simulink library "FAM_lab_scale_v3"  (R2024a)
settings: Solver=VariableStepAuto  StartTime=0.0  StopTime=10.0  RelTol=1e-3
undefined symbols (not defined in the file): FAM_elasticity, FAM_stretched_radius, FAM_unstretched_length, FAM_wall_thickness, fiber_angle_alpha, fiber_angle_alpha_unstr, hose_pump_force_enabled, hose_pump_max_stretch, hose_pump_throughFlow_adjust
settings Model: Creator=cmmcguir  LastModifiedBy=cmmcguir
settings RTWCC: GPUComputeCapability=3.5

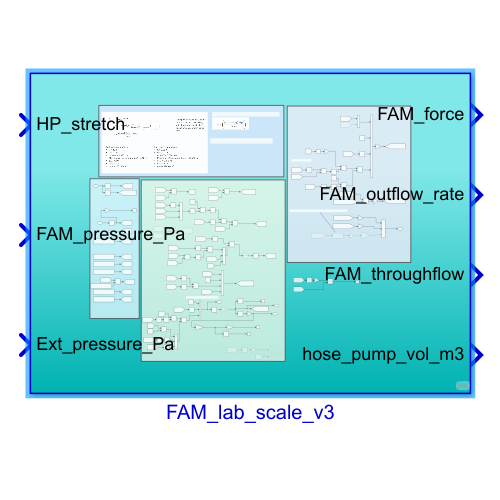
[thumbnail: Simulink's stored preview of the top-level diagram]
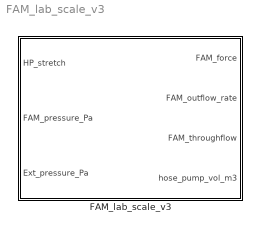
== system FAM_lab_scale_v3 ==
  FAM_lab_scale_v3 : Subsystem

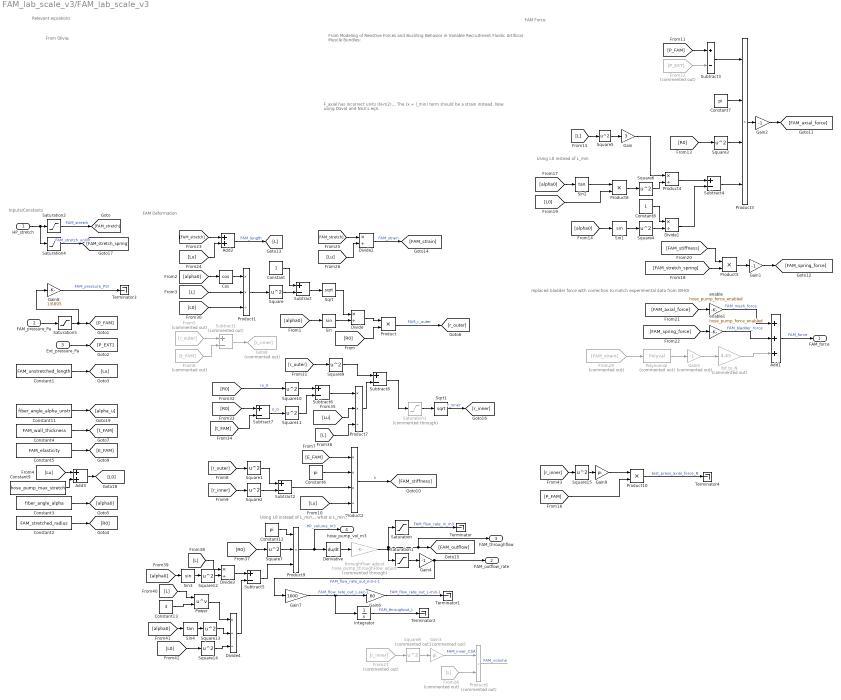
== system FAM_lab_scale_v3/FAM_lab_scale_v3 ==
  note: replaced bladder force with correction to match experimental data from WHOI
  note: F_axial has incorrect units (N-m2)... The (x + l_min) term should be a strain instead. Now using David and Nick's eqn.
  note: FAM Force
  note: Using L0 instead of L_min
  note: FAM Deformation
  note: Inputs/Constants
  note: Relevant equations
  note: From Modeling of Resistive Forces and Buckling Behavior in Variable Recruitment Fluidic Artificial Muscle Bundles:
  note: From Olivia:
  note: Using L0 instead of L_min... what is L_min?
  HP_stretch : Inport  Unit=m
  FAM_pressure_Pa : Inport  Port=2  Unit=Pa
  Ext_pressure_Pa : Inport  Port=3  Unit=Pa
  Add1 : Sum  Inputs=+++
  Add2 : Sum
  Add3 : Sum
  Constant : Constant
  Constant1 : Constant  Value=FAM_unstretched_length
  Constant11 : Constant  Value=fiber_angle_alpha_unstr
  Constant12 : Constant  Value=pi
  Constant13 : Constant  Value=3
  Constant2 : Constant  Value=FAM_stretched_radius
  Constant3 : Constant  Value=fiber_angle_alpha
  Constant4 : Constant  Value=FAM_wall_thickness
  Constant5 : Constant  Value=FAM_elasticity
  Constant6 : Constant  Value=pi
  Constant7 : Constant  Value=pi
  Constant8 : Constant
  Constant9 : Constant  Value=hose_pump_max_stretch
  Cos : Trigonometry  Operator=cos
  Derivative : Derivative
  Divide{,1..3} (4 alike) : Product  Inputs=*/
  Divide4 : Product  Inputs=*//
  From12 : From  Commented=on  GotoTag=P_EXT
  From27 : From  Commented=on  GotoTag=r_inner
  From28 : From  Commented=on  GotoTag=L
  From29 : From  Commented=on  GotoTag=FAM_strain
  From5 : From  Commented=on  GotoTag=r_outer
  From6 : From  Commented=on  GotoTag=t_FAM
  Gain : Gain  Gain=3
  Gain1 : Gain  Gain=-1
  Gain2 : Gain  Gain=-1
  Gain3 : Gain  Commented=on  Gain=pi
  Gain4 : Gain  Gain=-1
  Gain5 : Gain  Commented=on  Gain=-1
  Gain6 : Gain  Gain=60
  Gain7 : Gain  Gain=1000
  Gain8 : Gain  Gain=1/6895
  Gain9 : Gain  Gain=pi
  Goto8 : Goto  Commented=on  GotoTag=r_inner
  Integrator : Integrator
  Polynomial : Polyval  Commented=on  Coefs="1e5* [1.5724   -0.4144    0.0729   -0.0014]"
  Power : Math  Operator=pow
  Product{,5,8,10} (4 alike) : Product
  Product1 : Product  Inputs=**/
  Product2 : Product  Inputs=***/
  Product3 : Product  Inputs=****
  Product4 : Product  Inputs=*/
  Product6 : Product  Commented=on
  Product7 : Product  Inputs=**/
  Product9 : Product  Inputs=***
  Saturation : Saturate  UpperLimit=inf  LowerLimit=0  ZeroCross=off
  Saturation1 : Saturate  UpperLimit=0  LowerLimit=-inf  ZeroCross=off
  Saturation2 : Saturate  UpperLimit=hose_pump_max_stretch*1.5  LowerLimit=0
  Saturation3 : Saturate  Commented=through  UpperLimit=inf  LowerLimit=(FAM_wall_thickness*1.1)^2
  Saturation4 : Saturate  UpperLimit=inf  LowerLimit=0
  Saturation5 : Saturate  UpperLimit=inf  LowerLimit=0
  Sin : Trigonometry
  Sin1 : Trigonometry
  Sin2 : Trigonometry  Operator=tan
  Sin3 : Trigonometry
  Sin4 : Trigonometry  Operator=tan
  Sqrt : Sqrt
  Sqrt1 : Sqrt
  Square{,1..7,9..15} (15 alike) : Math  Operator=square
  Square8 : Math  Commented=on  Operator=square
  Subtract{,2..8} (8 alike) : Sum  Inputs=+-
  Subtract1 : Sum  Commented=on  Inputs=+-
  Terminator{,1..4} (5 alike) : Terminator
  enable : Gain  Gain=hose_pump_force_enabled
  enable1 : Gain  Gain=hose_pump_force_enabled
  lbf_to_N : Gain  Commented=on  Gain=4.45
  throughFlow_adjust : Gain  Commented=through  Gain=hose_pump_throughFlow_adjust
  FAM_force : Outport
  FAM_outflow_rate : Outport  Port=2
  FAM_throughflow : Outport  Port=3
  hose_pump_vol_m3 : Outport  Port=4
  wires:
  [FAM_stretch_spring] -> Product5/2
  [E_FAM] -> Product2/1
  [FAM_axial_force] -> enable/1
  [alpha0] -> Sin2/1
  Constant3/1 -> [alpha0]
  Gain/1 -> Product4/1
  [R0] -> Product/2
  Product2/1 -> [FAM_stiffness]  "k"
  From6/1 -> Subtract1/2
  Constant2/1 -> [R0]
  Ext_pressure_Pa/1 -> [P_EXT]
  [alpha0] -> Cos/1
  [FAM_stiffness] -> Product5/1
  Subtract2/1 -> Product2/3
  Product/1 -> [r_outer]  "FAM_r_outer"
  [alpha0] -> Sin1/1
  Product5/1 -> Gain1/1
  Constant4/1 -> [t_FAM]
  Square6/1 -> Product4/2
  Cos/1 -> Product1/1
  Product3/1 -> Gain2/1
  FAM_pressure_Pa/1 -> Saturation5/1
  Subtract/1 -> Sqrt/1
  Constant7/1 -> Product3/2
  [FAM_spring_force] -> enable1/1
  Constant/1 -> Subtract/1
  From12/1 -> Subtract3/2
  [Lu] -> Product2/4
  Add1/1 -> FAM_force/1  "FAM_force"
  Sin2/1 -> Product8/1
  [r_outer] -> Square1/1
  Product4/1 -> Subtract4/1
  Constant1/1 -> [Lu]
  Square/1 -> Subtract/2
  Constant6/1 -> Product2/2
  Divide1/1 -> Subtract4/2
  Subtract4/1 -> Product3/4
  Constant8/1 -> Divide1/1
  Divide/1 -> Product/1
  Sin1/1 -> Square4/1
  Subtract3/1 -> Product3/1
  Square3/1 -> Product3/3
  Square4/1 -> Divide1/2
  From5/1 -> Subtract1/1
  [P_FAM] -> Subtract3/1
  Subtract1/1 -> Goto8/1
  Sqrt/1 -> Divide/1
  [L] -> Product1/2
  Square1/1 -> Subtract2/1
  Product1/1 -> Square/1
  Constant5/1 -> [E_FAM]
  [R0] -> Square3/1
  Square2/1 -> Subtract2/2
  Sin/1 -> Divide/2
  [alpha0] -> Sin/1
  [r_inner] -> Square2/1
  Square5/1 -> Gain/1
  [L] -> Square5/1
  [FAM_stretch] -> Add2/1
  [Lu] -> Add2/2
  Add2/1 -> [L]  "FAM_length"
  Divide2/1 -> [FAM_strain]  "FAM_strain"
  [Lu] -> Divide2/2
  [FAM_stretch] -> Divide2/1
  Gain1/1 -> [FAM_spring_force]
  Gain2/1 -> [FAM_axial_force]
  Derivative/1 -> throughFlow_adjust/1
  Saturation/1 -> Terminator/1  "FAM_flow_rate_in_m3"
  Gain4/1 -> FAM_outflow_rate/1, Gain7/1  "FAM_flow_rate_out_m3-s-1"
  Saturation1/1 -> Gain4/1
  Gain6/1 -> Terminator1/1  "FAM_flow_rate_out_L-min-1"
  Gain7/1 -> Integrator/1, Gain6/1  "FAM_flow_rate_out_L-sec-1"
  Integrator/1 -> Terminator2/1  "FAM_throughput_L"
  Saturation2/1 -> [FAM_stretch]  "FAM_stretch"
  [r_outer] -> Square9/1
  [R0] -> Square10/1  "ro_0"
  Square10/1 -> Subtract6/1
  [R0] -> Subtract7/1
  [t_FAM] -> Subtract7/2
  Subtract7/1 -> Square11/1  "ri_0"
  Square11/1 -> Subtract6/2
  Subtract6/1 -> Product7/1
  [Lu] -> Product7/2
  Subtract8/1 -> Saturation3/1
  [L] -> Product7/3
  From29/1 -> Polynomial/1
  Polynomial/1 -> Gain5/1
  Gain5/1 -> lbf_to_N/1
  lbf_to_N/1 -> Add1/3
  Square9/1 -> Subtract8/1
  Product7/1 -> Subtract8/2
  HP_stretch/1 -> Saturation4/1, Saturation2/1
  Sqrt1/1 -> [r_inner]  "r_inner"
  Saturation3/1 -> Sqrt1/1
  Saturation4/1 -> [FAM_stretch_spring]  "FAM_stretch_unlim"
  Saturation5/1 -> Gain8/1, [P_FAM]
  Gain8/1 -> Terminator3/1  "FAM_pressure_PSI"
  Product8/1 -> Square6/1
  throughFlow_adjust/1 -> Saturation1/1, Saturation/1, FAM_throughflow/1, [FAM_outflow]
  enable/1 -> Add1/1  "FAM_mesh_force"
  enable1/1 -> Add1/2  "FAM_bladder_force"
  Constant9/1 -> Add3/2
  [Lu] -> Add3/1
  Add3/1 -> [L0]
  Constant11/1 -> [alpha_u]
  [L0] -> Product1/3
  Product6/1 -> ?  "FAM_volume"
  From27/1 -> Square8/1
  Square8/1 -> Gain3/1
  Gain3/1 -> Product6/1  "FAM_inner_CSA"
  From28/1 -> Product6/2
  Product9/1 -> hose_pump_vol_m3/1, Derivative/1  "HP_volume_m3"
  Constant12/1 -> Product9/1
  [R0] -> Square7/1
  Square7/1 -> Product9/2
  Subtract5/1 -> Product9/3
  Divide3/1 -> Subtract5/1
  Divide4/1 -> Subtract5/2
  [L] -> Divide3/1
  [alpha0] -> Sin3/1
  Square12/1 -> Divide3/2
  Sin3/1 -> Square12/1
  Sin4/1 -> Square13/1
  [alpha0] -> Sin4/1
  [L] -> Power/1
  Power/1 -> Divide4/1
  Square13/1 -> Divide4/2
  Constant13/1 -> Power/2
  [L0] -> Square14/1
  Square14/1 -> Divide4/3
  [L0] -> Product8/2
  [r_inner] -> Square15/1
  Square15/1 -> Gain9/1
  Gain9/1 -> Product10/1
  [P_FAM] -> Product10/2
  Product10/1 -> Terminator4/1  "test_press_axial_force_N"
